simulink model "testCycler"  (R2022a)
settings: Solver=VariableStepAuto  StartTime=0.0  StopTime=Inf  MaxStep=1e-3  RelTol=1e-3
undefined symbols (not defined in the file): Call, Function, Neg, Pos
libraries: fl_lib x4, nesl_utility x2, ee_lib x2
settings Model: Creator=mmarq  LastModifiedBy=mmarq

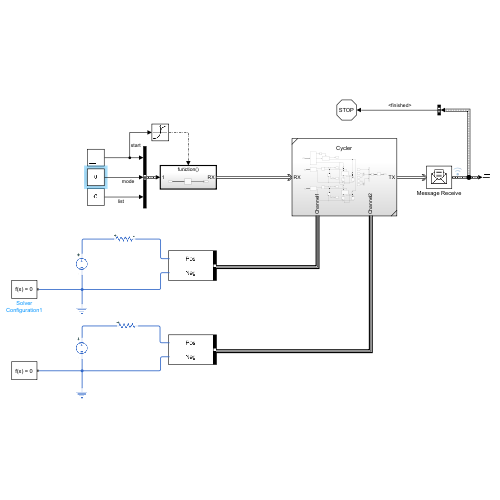
[thumbnail: Simulink's stored preview of the top-level diagram]
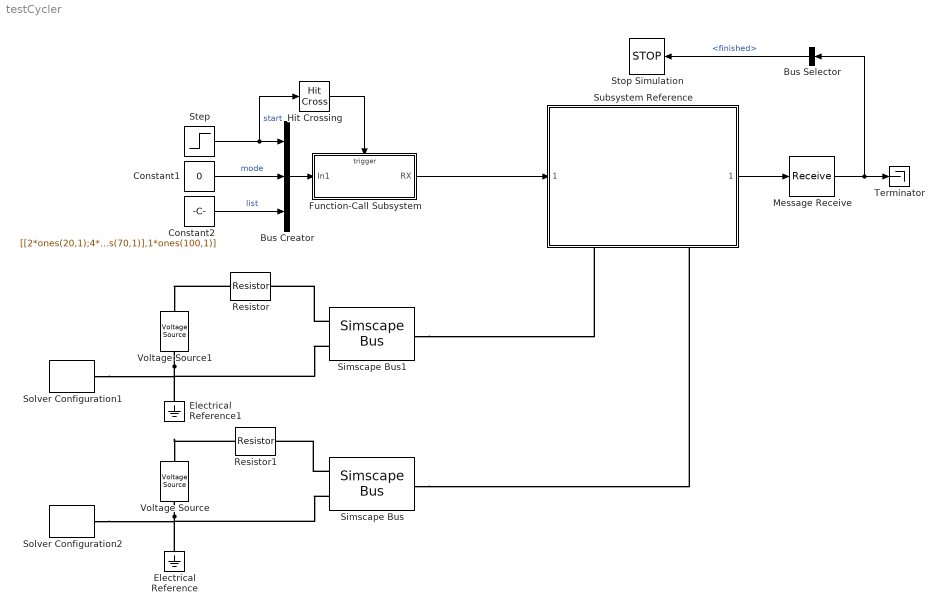
== system testCycler ==
  Bus Creator : BusCreator  Inputs=3  OutDataTypeStr=Bus: CyclerCmd  NonVirtualBus=on
      settings: InheritFromInputs=off
  Bus Selector : BusSelector  OutputSignals=finished
  Constant1 : Constant  Value=0
  Constant2 : Constant  Value=[[2*ones(20,1);4*ones(10,1);10*ones(70,1)],1*ones(100,1)]
  Electrical Reference : fl_lib/Electrical/Electrical Elements/Electrical Reference
      settings: SourceProductBaseCode=PW,SS,VE
  Electrical Reference1 : fl_lib/Electrical/Electrical Elements/Electrical Reference
      settings: SourceProductBaseCode=PW,SS,VE
  Function-Call Subsystem : Subsystem  TreatAsAtomicUnit=on
  Hit Crossing : HitCross  HitCrossingOffset=0.01  HitCrossingDirection=rising  HitCrossingOutputType=Function-Call
  Message Receive : Receive  InputPortMessageModes=m  ValueSourceWhenQueueIsEmpty=Use initial value
  Resistor : fl_lib/Electrical/Electrical Elements/Resistor  R=1 Ohm  i_specify=off  i_priority=None  i=0 A  i_nominal_specify=off  i_nominal_unit=A  i_nominal_value=1  v_specify=off  v_priority=None  v=0 V  v_nominal_specify=off  v_nominal_unit=V  v_nominal_value=1
      settings: SourceProductBaseCode=PW,SS,VE
  Resistor1 : fl_lib/Electrical/Electrical Elements/Resistor  R=1 Ohm  i_specify=off  i_priority=None  i=0 A  i_nominal_specify=off  i_nominal_unit=A  i_nominal_value=1  v_specify=off  v_priority=None  v=0 V  v_nominal_specify=off  v_nominal_unit=V  v_nominal_value=1
      settings: SourceProductBaseCode=PW,SS,VE
  Simscape Bus : SimscapeBus  HierarchyStrings=Pos;Neg
  Simscape Bus1 : SimscapeBus  HierarchyStrings=Pos;Neg
  Solver Configuration1 : nesl_utility/Solver Configuration  PhysicalDomain=network_engine_domain  SubClassName=solver  LeftPortType=input  RightPortType=generic  Tones=[]  Harmonics=[]  SimulateNoise=off  Profile=off  UseLocalSampling=off  EnableSwitchedLinearOptims=on  FrequencyDomain=off  UseCCode=off  RelTol=0.001  AbsTol=0.001  MinStep=1e-09  ToWorkspace=off  RevertToSquareIcSolve=off  NumHomotopyIterations=100  PhasorMode=off  PhasorModeNumHarmonics=1  IndexReductionMethod=DerivativeReplacement  DoDC=off  ResidualTolerance=1e-09  UseLocalSolver=off  LocalSolverChoice=NE_BACKWARD_EULER_ADVANCER  LocalSolverSampleTime=0.001  DoFixedCost=off  MaxNonlinIter=3  MaxModeIter=2  ComputeImpulses=off  ImpulseIterations=2  LinearAlgebra=auto  LinearAlgebraNumThread=0  EquationFormulation=NE_TIME_EF  DelaysMemoryBudget=1024  AutomaticFiltering=on  FilteringTimeConstant=0.001  PartitionStorageMethod=AS_NEEDED  PartitionMemoryBudget=1024  PartitionMethod=ROBUST
      settings: SourceProductBaseCode=SS,PW,VE
  Solver Configuration2 : nesl_utility/Solver Configuration  PhysicalDomain=network_engine_domain  SubClassName=solver  LeftPortType=input  RightPortType=generic  Tones=[]  Harmonics=[]  SimulateNoise=off  Profile=off  UseLocalSampling=off  EnableSwitchedLinearOptims=on  FrequencyDomain=off  UseCCode=off  RelTol=0.001  AbsTol=0.001  MinStep=1e-09  ToWorkspace=off  RevertToSquareIcSolve=off  NumHomotopyIterations=100  PhasorMode=off  PhasorModeNumHarmonics=1  IndexReductionMethod=DerivativeReplacement  DoDC=off  ResidualTolerance=1e-09  UseLocalSolver=off  LocalSolverChoice=NE_BACKWARD_EULER_ADVANCER  LocalSolverSampleTime=0.001  DoFixedCost=off  MaxNonlinIter=3  MaxModeIter=2  ComputeImpulses=off  ImpulseIterations=2  LinearAlgebra=auto  LinearAlgebraNumThread=0  EquationFormulation=NE_TIME_EF  DelaysMemoryBudget=1024  AutomaticFiltering=on  FilteringTimeConstant=0.001  PartitionStorageMethod=AS_NEEDED  PartitionMemoryBudget=1024  PartitionMethod=ROBUST
      settings: SourceProductBaseCode=SS,PW,VE
  Step : Step  SampleTime=0
  Stop Simulation : Stop
  Subsystem Reference : Subsystem  ReferencedSubsystem=Cycler
      settings: PortSchema="{\"entries\":[{\"content\":{\"sides\":[{\"content\":{\"connectorIds\":[\"In1\"]},\"type\":\"ConnectorPlacement.EquallySpacedRectSide\",\"uuid\":\"f71a85fa-5f1b-4f60-afc2-2af602cd6bfa\"},{\"content\":{\"connectorIds\":[\"Out1\"],\"side\":\"RIGHT\"},\"type\":\"ConnectorPlacement.EquallySpacedRectSide\",\"uuid\":\"a58ae27e-7fda-4e3b-bf34-5bf7de7a0120\"},{\"content\":{\"connectorIds\":[],\"side\":\"TOP\"},\"type\":\"ConnectorPlacement.EquallySpacedRectSide\",\"uuid\":\"cf49a94a-a45d-4ba1-8d31-8fa348aa4236\"},{\"content\":{\"connectorIds\":[\"LConn1\",\"LConn2\"],\"side\":\"BOTTOM\"},\"type\":\"ConnectorPlacement.EquallySpacedRectSide\",\"uuid\":\"bc55b36a-d3dc-4da8-86e8-8e6c8b2be31d\"}]},\"type\":\"ConnectorPlacement.EquallySpacedConnector\",\"uuid\":\"5fb0b0ec-3310-4f5c-9c9c-9e0d49a0c2e5\"}],\"packageUris\":[\"http://schema.mathworks.com/mf0/Connector/R2020b\"],\"version\":\"1.0\"}"
  Terminator : Terminator
  Voltage Source : ee_lib/Sources/Voltage Source  dc_voltage=15 V  ac_voltage=0 V  ac_shift=0 rad  ac_frequency=60 Hz  noise_mode=0  PSD=0 V^2/Hz  repeatability=1  auto_seed=3499211588  user_seed=0  sample_time=1e-3 s  i_specify=off  i_priority=None  i=0 A  i_nominal_specify=off  i_nominal_unit=A  i_nominal_value=1  v_specify=off  v_priority=None  v=0 V  v_nominal_specify=off  v_nominal_unit=V  v_nominal_value=1
  Voltage Source1 : ee_lib/Sources/Voltage Source  dc_voltage=15 V  ac_voltage=0 V  ac_shift=0 rad  ac_frequency=60 Hz  noise_mode=0  PSD=0 V^2/Hz  repeatability=1  auto_seed=3890346746  user_seed=0  sample_time=1e-3 s  i_specify=off  i_priority=None  i=0 A  i_nominal_specify=off  i_nominal_unit=A  i_nominal_value=1  v_specify=off  v_priority=None  v=0 V  v_nominal_specify=off  v_nominal_unit=V  v_nominal_value=1
  wires:
  Hit Crossing/1 -> Function-Call Subsystem/Trigger
  Constant2/1 -> Bus Creator/3  "list"
  Step/1 -> Hit Crossing/1, Bus Creator/1  "start"
  Constant1/1 -> Bus Creator/2  "mode"
  Bus Creator/1 -> Function-Call Subsystem/1(In1)
  Function-Call Subsystem/1(RX) -> Subsystem Reference/1
  Subsystem Reference/1 -> Message Receive/1
  Bus Selector/1 -> Stop Simulation/1  "<finished>"
  Message Receive/1 -> Bus Selector/1, Terminator/1
  connections:
  Voltage Source/RConn1 -- Simscape Bus/LConn2 -- Solver Configuration2/RConn1 -- Electrical Reference/LConn1
  Voltage Source1/RConn1 -- Solver Configuration1/RConn1 -- Simscape Bus1/LConn2 -- Electrical Reference1/LConn1
  Simscape Bus1/RConn1 -- Subsystem Reference/LConn1
  Resistor/LConn1 -- Voltage Source1/LConn1
  Simscape Bus/RConn1 -- Subsystem Reference/LConn2
  Simscape Bus/LConn1 -- Resistor1/RConn1
  Simscape Bus1/LConn1 -- Resistor/RConn1
  Resistor1/LConn1 -- Voltage Source/LConn1

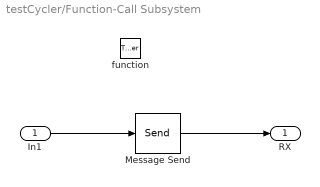
== system testCycler/Function-Call Subsystem ==
  In1 : Inport
  function : TriggerPort  TriggerType=function-call  VariantControl=(inherit)
  Message Send : Send  OutputPortMessageModes=m
  RX : Outport
  wires:
  In1/1 -> Message Send/1
  Message Send/1 -> RX/1
